simulink model "psbparalbranch"  (Simulink 6.0)
settings: Solver=ode23s  SolverMode=SingleTasking  StartTime=0.0  StopTime=0.1  RelTol=1e-3  AbsTol=1e-6
libraries: powerlib2 x6
settings Model: Creator=patrice  LastModifiedBy=batserve  ExtModeTrigMode=oneshot  ExtModeArmWhenConnect=off  ExtModeAutoUpdateStatusClock=off
settings DataIOCC: LimitDataPoints=off
settings OptimizationCC: BooleanDataType=off
settings DebuggingCC: SolverPrmCheckMsg=none
settings HardwareCC: TargetUnknown=on
settings RTWCC: TemplateMakefile=grt_unix.tmf

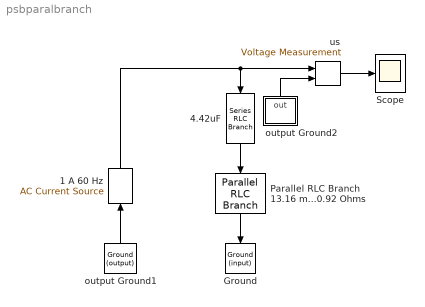
== system psbparalbranch ==
  1 A 60 Hz : powerlib2/Electrical Sources/AC Current Source  Tag=PoWeRsYsTeMbLoCk  Orientation=up  A=1  P=0  F=60  stime=0  mesure=None  PSBOutputType=1
  4.42uF : powerlib2/Elements/Series RLC Branch  Tag=PoWeRsYsTeMbLoCk  Orientation=down  a=0  b=0  c=4.42e-06  mesure=None  PSBOutputType=1
  Ground : powerlib2/Connectors/Ground (input)  Tag=PoWeRsYsTeMbLoCk  Orientation=down
  Parallel RLC Branch 13.16 mH  70.92 Ohms : powerlib2/Elements/Parallel RLC Branch  Tag=PoWeRsYsTeMbLoCk  Orientation=down  a=70.92  b=13.16e-03  c=0  mesure=None  PSBOutputType=1
  Scope : Scope
      settings: TickLabels=on  TimeRange=0.1  YMin=-1000  YMax=1000  DataFormat=Array
  output Ground1 : powerlib2/Connectors/Ground (output)  Tag=PoWeRsYsTeMbLoCk  Orientation=up  PSBOutputType=1
  output Ground2 : Subsystem  Tag=PoWeRsYsTeMbLoCk  Orientation=up
      mask Type: Ground
      mask Description: Ground connexion
      mask Help: web(psbhelp);
      mask Display: plot(-15,-15,15,15,[5 5],[-10 10],[0 0],[-5 5],[-5 -5],[-2.5 2.5],[15 5],[0 0])
  us : powerlib2/Measurements/Voltage Measurement  Tag=PoWeRsYsTeMmEaSuReMeNt  PSBOutputType=0  PSBequivalent=1
  wires:
  us/1 -> Scope/1
  output Ground2/1(out) -> us/2
  1 A 60 Hz/1 -> 4.42uF/1, us/1
  4.42uF/1 -> Parallel RLC Branch 13.16 mH  70.92 Ohms/1
  Parallel RLC Branch 13.16 mH  70.92 Ohms/1 -> Ground/1
  output Ground1/1 -> 1 A 60 Hz/1

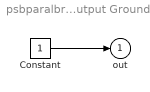
== system psbparalbranch/output Ground2 ==
  Constant : Constant
  out : Outport  InitialOutput=0
  wires:
  Constant/1 -> out/1
